simulink model "danxiangtiaoya"  (R2015b)
settings: Solver=ode15s  StartTime=0.0  StopTime=0.04  RelTol=1e-3
libraries: powerlib x8
settings Model: Creator=Administrator  LastModifiedBy=Administrator
settings DataIOCC: SaveFormat=Array  SignalLoggingSaveFormat=ModelDataLogs  SaveOutput=off  SaveTime=off
settings OptimizationCC: BooleanDataType=off  InitFltsAndDblsToZero=on
settings DebuggingCC: SaveWithParameterizedLinksMsg=none  UnderspecifiedInitializationDetection=Classic  MergeDetectMultiDrivingBlocksExec=none  SignalResolutionControl=TryResolveAllWithWarning  MultiTaskDSMMsg=warning  MultiTaskCondExecSysMsg=none  FcnCallInpInsideContextMsg=UseLocalSettings
settings HardwareCC: ProdBitPerPointer=32  ProdLargestAtomicFloat=None  ProdIntDivRoundTo=Undefined  ProdEndianess=Unspecified  ProdWordSize=32  ProdHWDeviceType=32-bit Generic  TargetUnknown=on
settings GRTTargetCC: TargetFcnLib=ansi_tfl_tmw.mat  CombineOutputUpdateFcns=off  GRTInterface=on
settings ConfigComp: CovModelRefEnable=Off

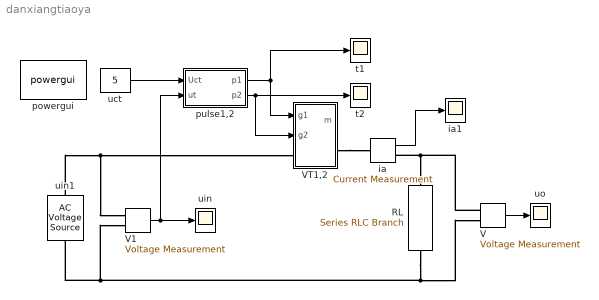
== system danxiangtiaoya ==
  RL : powerlib/Elements/Series RLC Branch  LConnTagsString=__new0  RConnTagsString=__new0  BranchType=RL  Resistance=1  Inductance=1e-3  SetiL0=off  InitialCurrent=0  Capacitance=[]  Setx0=off  InitialVoltage=0  Measurements=None
  V : powerlib/Measurements/Voltage Measurement  PhasorSimulation=off  OutputType=Magnitude  PSBequivalent=0
  V1 : powerlib/Measurements/Voltage Measurement  PhasorSimulation=off  OutputType=Magnitude  PSBequivalent=0
  VT1,2 : Subsystem
  ia : powerlib/Measurements/Current Measurement  PhasorSimulation=off  OutputType=Magnitude  PSBequivalent=0
  ia1 : Scope
  powergui : powerlib/powergui  Priority=1  SimulationMode=Continuous  SolverType=Tustin/Backward Euler (TBE)  SampleTime=50e-6  frequency=60  SPID=off  DisableSnubberDevices=off  DisableRonSwitches=off  DisableVfSwitches=off  SwTol=0  DisplayEquations=off  Interpol=off  ExternalGateDelay=off  methode=off  Ts=10  FunctionMessages=off  echomessages=off  HookPort=off  EnableUseOfTLC=off  x0status=blocks  frequencyindice=50  Pbase=100e6  ErrMax=1e-4  Iterations=50  UnitsV=kV  UnitsW=MW  buscounter=0  RestoreLinks=warning  ResistiveCurrentMeasurement=off  Frange=[0:2:500]  Ylog=off  Xlog=on  ShowGrid=off  save=off  variable=ZData  structure=0  ZoomFFT=off  StartTime=0.0  cycles=1  DisplayStyle=1  fundamental=60  FreqAxis=off  MaxFrequency=1000  frequencyindicesteady=1  RmsSteady=1  display=off
  pulse1,2 : Subsystem
  t1 : Scope
  t2 : Scope
  uct : Constant  Value=5
  uin : Scope
  uin1 : powerlib/Electrical Sources/AC Voltage Source  Amplitude=220  Phase=0  Frequency=50  SampleTime=0  Measurements=None  BusType=swing  Pref=10e3  Qref=0  Qmin=-inf  Qmax=+inf
  uo : Scope
  wires:
  V/1 -> uo/1
  ia/1 -> ia1/1
  pulse1,2/1(p1) -> t1/1, VT1,2/1(g1)
  pulse1,2/2(p2) -> t2/1, VT1,2/2(g2)
  uct/1 -> pulse1,2/1(Uct)
  V1/1 -> uin/1, pulse1,2/2(ut)
  connections:
  uin1/RConn1 -- VT1,2/LConn1 -- V1/LConn1
  RL/RConn1 -- V/LConn2 -- uin1/LConn1 -- V1/LConn2
  V/LConn1 -- ia/RConn1 -- RL/LConn1
  VT1,2/RConn1 -- ia/LConn1

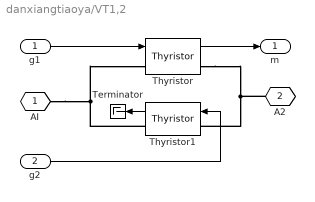
== system danxiangtiaoya/VT1,2 ==
  g1 : Inport
  g2 : Inport  Port=2
  Terminator : Terminator
  Thyristor : powerlib/Power Electronics/Thyristor  Ron=1e-03  Lon=0  Vf=0.8  IC=0  Rs=1000  Cs=inf  Measurements=on
  Thyristor1 : powerlib/Power Electronics/Thyristor  Ron=1e-03  Lon=0  Vf=0.8  IC=0  Rs=1000  Cs=inf  Measurements=on
  AI : PMIOPort  Tag=PMCPort  Port=1  Side=Left
  A2 : PMIOPort  Tag=PMCPort  Port=2  Side=Right
  m : Outport
  wires:
  g1/1 -> Thyristor/1
  g2/1 -> Thyristor1/1
  Thyristor/1 -> m/1
  Thyristor1/1 -> Terminator/1
  connections:
  Thyristor1/RConn1 -- Thyristor/LConn1 -- AI/RConn1
  Thyristor/RConn1 -- Thyristor1/LConn1 -- A2/RConn1

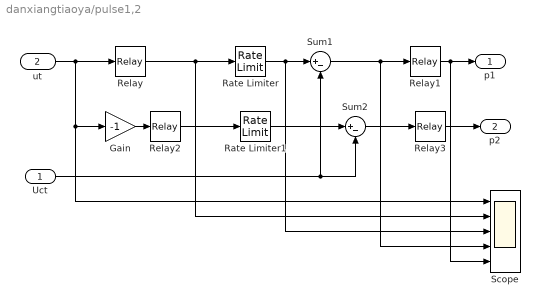
== system danxiangtiaoya/pulse1,2 ==
  Uct : Inport
  ut : Inport  Port=2
  Gain : Gain  Gain=-1  SaturateOnIntegerOverflow=on  OutDataTypeStr=Inherit: Same as input  ParamDataTypeStr=Inherit: Same as input
  Rate Limiter : RateLimiter  RisingSlewLimit=1000  FallingSlewLimit=-1e8
  Rate Limiter1 : RateLimiter  RisingSlewLimit=1000  FallingSlewLimit=-1e8
  Relay : Relay  OnOutputValue=10
  Relay1 : Relay
  Relay2 : Relay  OnOutputValue=10
  Relay3 : Relay
  Scope : Scope  NumInputPorts=5
  Sum1 : Sum  Inputs=|+-  SaturateOnIntegerOverflow=on  InputSameDT=on  OutDataTypeStr=Inherit: Same as first input
  Sum2 : Sum  Inputs=|+-  SaturateOnIntegerOverflow=on  InputSameDT=on  OutDataTypeStr=Inherit: Same as first input
  p1 : Outport
  p2 : Outport  Port=2
  wires:
  Relay/1 -> Rate Limiter/1, Scope/2
  Rate Limiter/1 -> Sum1/1, Scope/3
  Sum1/1 -> Relay1/1, Scope/4
  Gain/1 -> Relay2/1
  Rate Limiter1/1 -> Sum2/1
  Sum2/1 -> Relay3/1
  Relay2/1 -> Rate Limiter1/1
  Relay1/1 -> p1/1, Scope/5
  Relay3/1 -> p2/1
  ut/1 -> Relay/1, Gain/1, Scope/1
  Uct/1 -> Sum2/2, Sum1/2
